simulink model "read_uart"  (R2014b)
settings: Solver=ode45  StartTime=0.0  StopTime=10.0  RelTol=1e-3
libraries: ec_arm_cortex_a_lib x1
settings Model: Creator=Michael  LastModifiedBy=Michael
settings RTWCC: CustomSourceCode="#include \"increment.cpp\""  CustomHeaderCode="#include \"increment.h\""  CustomInclude=$/custom_c_code

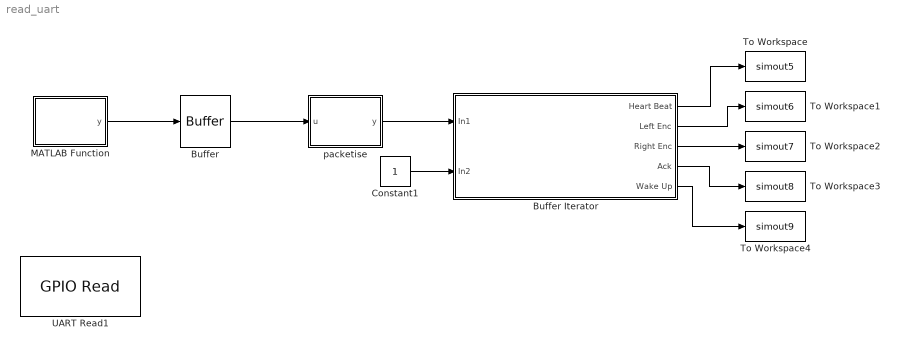
== system read_uart ==
  Buffer : Buffer  N=255  TreatMby1Signals=One channel
  "Buffer Iterator " : Subsystem
  Constant1 : Constant  OutDataTypeStr=uint8
  MATLAB Function : MATLAB Function  TreatAsAtomicUnit=on
  To Workspace : ToWorkspace  VariableName=simout5  SaveFormat=Timeseries  SampleTime=-1
  To Workspace1 : ToWorkspace  VariableName=simout6  SaveFormat=Timeseries  SampleTime=-1
  To Workspace2 : ToWorkspace  VariableName=simout7  SaveFormat=Timeseries  SampleTime=-1
  To Workspace3 : ToWorkspace  VariableName=simout8  SaveFormat=Timeseries  SampleTime=-1
  To Workspace4 : ToWorkspace  VariableName=simout9  SaveFormat=Timeseries  SampleTime=-1
  UART Read1 : ec_arm_cortex_a_lib/GPIO Read  board=BeagleBone Black  gpio=P9_11  internalResistor=None  sampleTime=1/115200  direction=Input  blockPlatform=BeagleBone
  packetise : MATLAB Function  TreatAsAtomicUnit=on
  wires:
  packetise/1(y) -> "Buffer Iterator "/1(In1)
  Constant1/1 -> "Buffer Iterator "/2(In2)
  Buffer/1 -> packetise/1(u)
  "Buffer Iterator "/1(Heart Beat) -> To Workspace/1
  "Buffer Iterator "/2(Left Enc) -> To Workspace1/1
  "Buffer Iterator "/3(Right Enc) -> To Workspace2/1
  "Buffer Iterator "/4(Ack) -> To Workspace3/1
  "Buffer Iterator "/5(Wake Up) -> To Workspace4/1
  MATLAB Function/1(y) -> Buffer/1

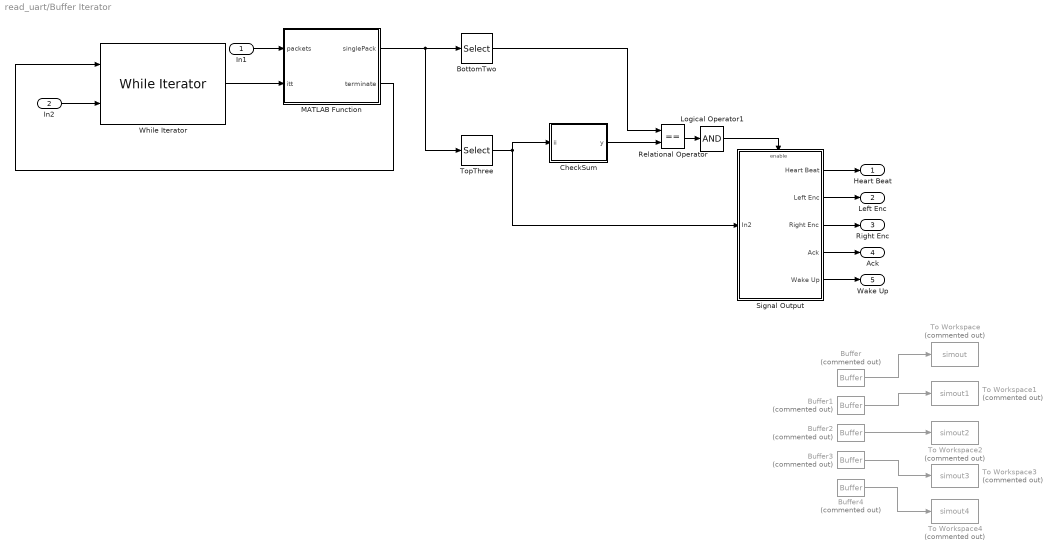
== system read_uart/Buffer Iterator  ==
  In1 : Inport
  In2 : Inport  Port=2  OutDataTypeStr=uint8
  BottomTwo : Selector  InputPortWidth=5  Indices=[4:5]  OutputSizes=2
  Buffer{,1..4} (5 alike) : Buffer  Commented=on  TreatMby1Signals=One channel
  CheckSum : MATLAB Function  TreatAsAtomicUnit=on
  Logical Operator1 : Logic  Inputs=1  AllPortsSameDT=off  OutDataTypeStr=boolean
  MATLAB Function : MATLAB Function  TreatAsAtomicUnit=on
  Relational Operator : RelationalOperator  Operator===  OutDataTypeStr=boolean
  Signal Output : Subsystem
  To Workspace : ToWorkspace  Commented=on  VariableName=simout  SaveFormat=Timeseries  SampleTime=-1
  To Workspace1 : ToWorkspace  Commented=on  VariableName=simout1  SaveFormat=Timeseries  SampleTime=-1
  To Workspace2 : ToWorkspace  Commented=on  VariableName=simout2  SaveFormat=Timeseries  SampleTime=-1
  To Workspace3 : ToWorkspace  Commented=on  VariableName=simout3  SaveFormat=Timeseries  SampleTime=-1
  To Workspace4 : ToWorkspace  Commented=on  VariableName=simout4  SaveFormat=Timeseries  SampleTime=-1
  TopThree : Selector  InputPortWidth=5  Indices=[1:3]
  While Iterator : WhileIterator  MaxIters=-1  ResetStates=reset  ShowIterationPort=on  OutputDataType=int8
  Heart Beat : Outport
  Left Enc : Outport  Port=2
  Right Enc : Outport  Port=3
  Ack : Outport  Port=4
  Wake Up : Outport  Port=5
  wires:
  In1/1 -> MATLAB Function/1(packets)
  While Iterator/1 -> MATLAB Function/2(itt)
  TopThree/1 -> Signal Output/1(In2), CheckSum/1(ii)
  BottomTwo/1 -> Relational Operator/1
  CheckSum/1(y) -> Relational Operator/2
  MATLAB Function/1(singlePack) -> TopThree/1, BottomTwo/1
  MATLAB Function/2(terminate) -> While Iterator/1
  Relational Operator/1 -> Logical Operator1/1
  In2/1 -> While Iterator/2
  Logical Operator1/1 -> Signal Output/Enable
  Signal Output/1(Heart Beat) -> Heart Beat/1
  Buffer/1 -> To Workspace/1
  Buffer1/1 -> To Workspace1/1
  Buffer2/1 -> To Workspace2/1
  Buffer3/1 -> To Workspace3/1
  Buffer4/1 -> To Workspace4/1
  Signal Output/2(Left Enc) -> Left Enc/1
  Signal Output/3(Right Enc) -> Right Enc/1
  Signal Output/4(Ack) -> Ack/1
  Signal Output/5(Wake Up) -> Wake Up/1

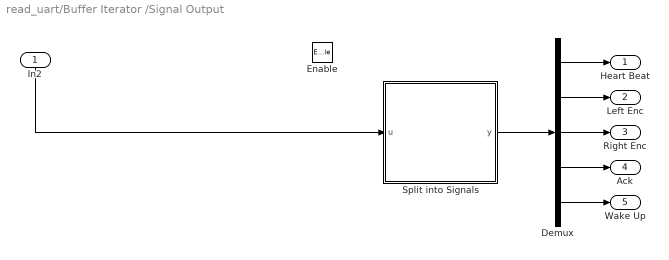
== system read_uart/Buffer Iterator /Signal Output ==
  In2 : Inport
  Enable : EnablePort
  Demux : Demux  Outputs=5
  Split into Signals : MATLAB Function  TreatAsAtomicUnit=on
  Heart Beat : Outport
  Left Enc : Outport  Port=2
  Right Enc : Outport  Port=3
  Ack : Outport  Port=4
  Wake Up : Outport  Port=5
  wires:
  In2/1 -> Split into Signals/1(u)
  Split into Signals/1(y) -> Demux/1
  Demux/5 -> Wake Up/1
  Demux/4 -> Ack/1
  Demux/3 -> Right Enc/1
  Demux/1 -> Heart Beat/1
  Demux/2 -> Left Enc/1

== matlab function read_uart/Buffer Iterator /CheckSum ==
  data: ii input; y output
function y = fletcher16(ii)
%#codegen

sum1 = uint16(0);
sum2 = uint16(0);

% Sum over all elements, modding by 255
for index = 1:length(ii)
   sum1 = mod(sum1 + uint16(ii(index)), 255);
   sum2 = mod(sum1 + sum2, 255);
end

% Fill empty uint8 array
y = [0; 0];

y(1) = uint8(255 - mod(sum1 + sum2, 255));
y(2) = uint8(255 - mod(sum1 + y(1), 255));

return;
% Finished

== matlab function read_uart/packetise ==
  data: u input uint8 size=[255 1]; y output Bus: PacketsBus [0..255]
function y = packetise(u)
%#codegen
assert (length(u) <= 255 );

persistent buffer;
persistent buf_len;

% Input is a binary string. We need to parse

if isempty(buffer)
    buffer = zeros(4,1,'uint8');
end

if isempty(buf_len)
    buf_len = 0;
end

% Prepend our previous buffer if it has a value
if buf_len > 0
    current_buffer = uint8([buffer(1:buf_len) u']);
else
    current_buffer = uint8(u);
end

rows = floor(length(current_buffer)/40);
assert(rows <= 51);

y.cmd=zeros(rows,1,'uint8');
y.id=zeros(rows,1,'uint8');
y.data=zeros(rows,1,'uint8');
y.c0=zeros(rows,1,'uint8');
y.c1=zeros(rows,1,'uint8');

for index = 1:rows
    y.cmd(index)=u((index-1)*5+1);
    y.id(index)=u((index-1)*5+2);
    y.data(index)=u((index-1)*5+3);
    y.c0(index)=u((index-1)*5+4);
    y.c1(index)=u((index-1)*5+5);
end

buf_len = mod(length(current_buffer), 5);
if buf_len > 0
    buffer(1:buf_len) = u((length(u)+1-buf_len) :length(u))';
end

== matlab function read_uart/Buffer Iterator /Signal Output/Split into Signals ==
  data: u input; y output
function y = parse_packet(u)
%#codegen

% y is an array of size 5, for the 5 possible data outputs
y = uint8(zeros(5,1));

% Decide what to do based on the command packet:
switch u(1)
    % Heart Beat
    case 1
        y(1) = u(2);
        return;
    % Left Encoder Data
    case 2
        y(2) = u(3);
        y(4) = u(2);
        return;
    % Right Encoder Data
    case 4
        y(3) = u(3);
        y(4) = u(2);
        return;
    % Wake Up
    case 16
        y(5) = u(2);
        return;
    % Acknowledge / All else
    case 8
        return
        % Nop
end

== matlab function read_uart/Buffer Iterator /MATLAB Function ==
  data: packets input Bus: PacketsBus; itt input; singlePack output uint8 size=[5 1]; terminate output
function [singlePack, terminate] = select_row(packets, itt)
%#codegen
terminate=logical(1);
singlePack=zeros(5,1,'uint8');

if length(packets.cmd) < itt
    terminate = logical(0);
    return;
end

if ~isempty(packets.cmd(itt))
    singlePack=[packets.cmd(itt); packets.id(itt); packets.data(itt); packets.c0(itt); packets.c1(itt) ];
end

== matlab function read_uart/MATLAB Function ==
  data: y output
function y = get_number
%#codegen
y = uint8(0);
y = get_number();
%y = coder.ceval('get_number');
